simulink model "untitled"  (R2012b)
settings: Solver=ode45  StartTime=0.0  StopTime=1  RelTol=1e-5
settings Model: Creator=Augusto  LastModifiedBy=Augusto

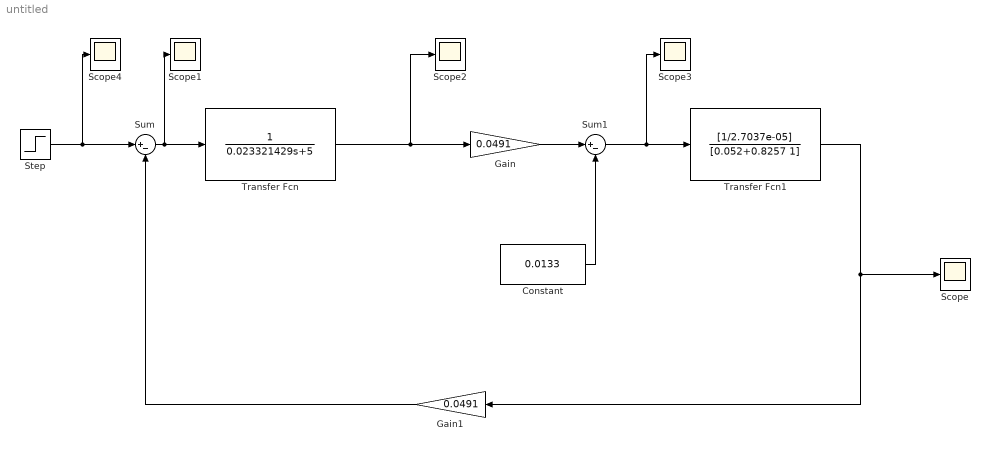
== system untitled ==
  Constant : Constant  Value=0.0133
  Gain : Gain  Gain=0.0491
  Gain1 : Gain  Gain=0.0491
  Scope{,1..4} (5 alike) : Scope
      Scope2 settings: SaveName=ScopeData2
      Scope3 settings: SaveName=ScopeData3
      Scope4 settings: SaveName=ScopeData4
  Step : Step  Time=0  After=5  SampleTime=0
  Sum : Sum  Inputs=|+-
  Sum1 : Sum  Inputs=|+-
  Transfer Fcn : TransferFcn  Denominator=[0.023321429 5]
  Transfer Fcn1 : TransferFcn  Numerator=[1/2.7037e-05]  Denominator=[0.052+0.8257 1]
  wires:
  Step/1 -> Scope4/1, Sum/1
  Gain/1 -> Sum1/1
  Sum1/1 -> Scope3/1, Transfer Fcn1/1
  Constant/1 -> Sum1/2
  Gain1/1 -> Sum/2
  Transfer Fcn1/1 -> Scope/1, Gain1/1
  Transfer Fcn/1 -> Scope2/1, Gain/1
  Sum/1 -> Scope1/1, Transfer Fcn/1
